simulink model "NL_Before_PLA"  (R2019b)
settings: Solver=VariableStepAuto  StartTime=0.0  StopTime=testtime  RelTol=1e-3
InitFcn:
  | NL_Before_PLA_Test_Parameters
StopFcn:
  | Verify_NL_Before_PLA
values from neighbouring files (symbols this model uses):
  cf_factor = min(cfsat, 10^(cfslope*cf/1e3 + cfconst)) * 2.0    [NL_Before_PLA_Test_Parameters.m]
  Fs = 48e3    (= 48000)    [NL_Before_PLA_Test_Parameters.m]
  multFac = max(2.95*max(1.0,1.5-spont/100), 4.3-0.2*cf/1e3)    [NL_Before_PLA_Test_Parameters.m]
  spont = 100    [NL_Before_PLA_Test_Parameters.m]
libraries: dspsrcs4 x2, simulink x1
settings Model: Creator=mblun  LastModifiedBy=t96f346
settings SFSimCC: CustomCodeUndefinedFunction=UseInterfaceOnly

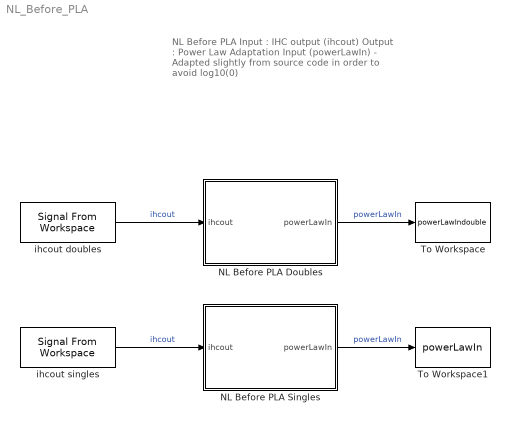
== system NL_Before_PLA ==
  note: NL Before PLA
      |
      | Input : IHC output (ihcout)
      |
      | Output : Power Law Adaptation Input (powerLawIn)
      |
      | - Adapted slightly from source code in order to avoid log10(0)
  NL Before PLA Doubles : Subsystem
  NL Before PLA Singles : Subsystem
  To Workspace : ToWorkspace  VariableName=powerLawIndouble  SampleTime=-1
      settings: Save2DSignal=2-D array (concatenate along first dimension)
  To Workspace1 : ToWorkspace  VariableName=powerLawIn  SampleTime=-1
      settings: Save2DSignal=2-D array (concatenate along first dimension)
  "ihcout doubles " : dspsrcs4/Signal From Workspace  X=RxSignalDouble  Ts=1/Fs  nsamps=1  OutputAfterFinalValue=Setting to zero  ignoreOrWarnInputAndFrameLengths=off  OutputFrames=off
  ihcout singles : dspsrcs4/Signal From Workspace  X=RxSignal  Ts=1/Fs  nsamps=1  OutputAfterFinalValue=Setting to zero  ignoreOrWarnInputAndFrameLengths=off  OutputFrames=off
  wires:
  NL Before PLA Doubles/1(powerLawIn) -> To Workspace/1  "powerLawIn"
  "ihcout doubles "/1 -> NL Before PLA Doubles/1(ihcout)  "ihcout"
  ihcout singles/1 -> NL Before PLA Singles/1(ihcout)  "ihcout"
  NL Before PLA Singles/1(powerLawIn) -> To Workspace1/1  "powerLawIn"

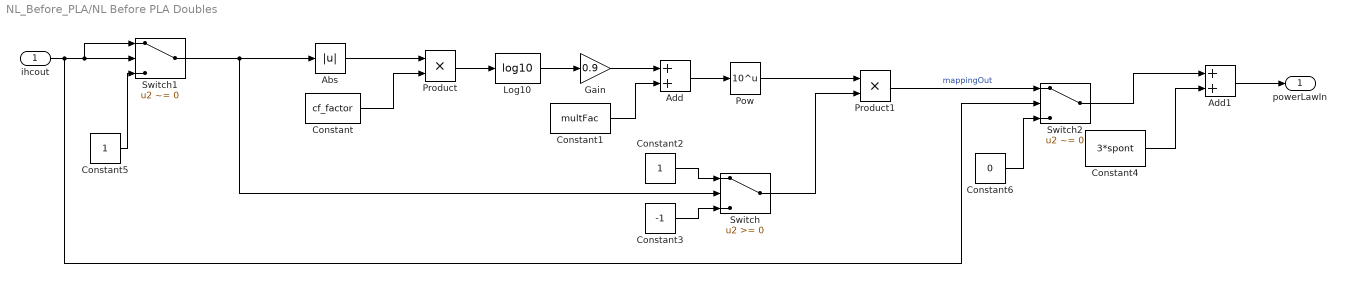
== system NL_Before_PLA/NL Before PLA Doubles ==
  ihcout : Inport
  Abs : Abs
  Add : Sum
  Add1 : Sum
  Constant : Constant  Value=cf_factor  SampleTime=-1
  Constant1 : Constant  Value=multFac  SampleTime=-1
  Constant2 : Constant  SampleTime=-1
  Constant3 : Constant  Value=-1  SampleTime=-1
  Constant4 : Constant  Value=3*spont  SampleTime=-1
  Constant5 : Constant  SampleTime=-1
  Constant6 : Constant  Value=0  SampleTime=-1
  Gain : Gain  Gain=0.9
  Log10 : Math  Operator=log10  RndMeth=Zero  SaturateOnIntegerOverflow=on
  Pow : Math  Operator=10^u  RndMeth=Zero  SaturateOnIntegerOverflow=on
  Product : Product
  Product1 : Product
  Switch : Switch
  Switch1 : Switch  Criteria=u2 ~= 0  ZeroCross=off
  Switch2 : Switch  Criteria=u2 ~= 0  ZeroCross=off
  powerLawIn : Outport  VectorParamsAs1DForOutWhenUnconnected=off
  wires:
  Switch1/1 -> Switch/2, Abs/1
  Constant/1 -> Product/2
  Abs/1 -> Product/1
  Product/1 -> Log10/1
  Log10/1 -> Gain/1
  Gain/1 -> Add/1
  Constant1/1 -> Add/2
  Add/1 -> Pow/1
  Constant3/1 -> Switch/3
  Constant2/1 -> Switch/1
  Pow/1 -> Product1/1
  Switch/1 -> Product1/2
  Constant4/1 -> Add1/2
  Add1/1 -> powerLawIn/1
  ihcout/1 -> Switch2/2, Switch1/1, Switch1/2
  Constant6/1 -> Switch2/3
  Switch2/1 -> Add1/1
  Constant5/1 -> Switch1/3
  Product1/1 -> Switch2/1  "mappingOut"

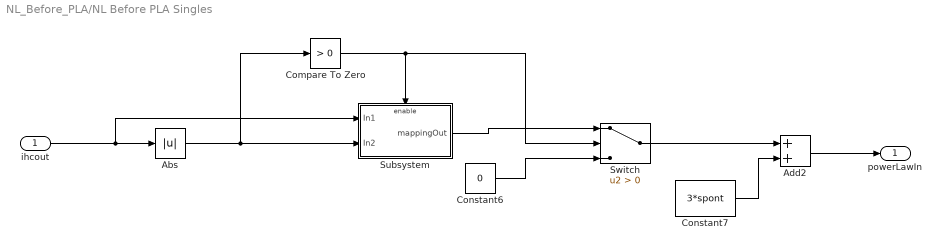
== system NL_Before_PLA/NL Before PLA Singles ==
  ihcout : Inport
  Abs : Abs
  Add2 : Sum
  Compare To Zero : simulink/Logic and Bit Operations/Compare To Zero  relop=>  OutDataTypeStr=boolean
  Constant6 : Constant  Value=0  OutDataTypeStr=single  SampleTime=-1
  Constant7 : Constant  Value=3*spont  OutDataTypeStr=single  SampleTime=-1
  Subsystem : Subsystem
  Switch : Switch  Criteria=u2 > Threshold  OutDataTypeStr=single
  powerLawIn : Outport  VectorParamsAs1DForOutWhenUnconnected=off
  wires:
  Constant6/1 -> Switch/3
  Switch/1 -> Add2/1
  Constant7/1 -> Add2/2
  Add2/1 -> powerLawIn/1
  ihcout/1 -> Subsystem/1(In1), Abs/1
  Abs/1 -> Compare To Zero/1, Subsystem/2(In2)
  Subsystem/1(mappingOut) -> Switch/1
  Compare To Zero/1 -> Subsystem/Enable, Switch/2

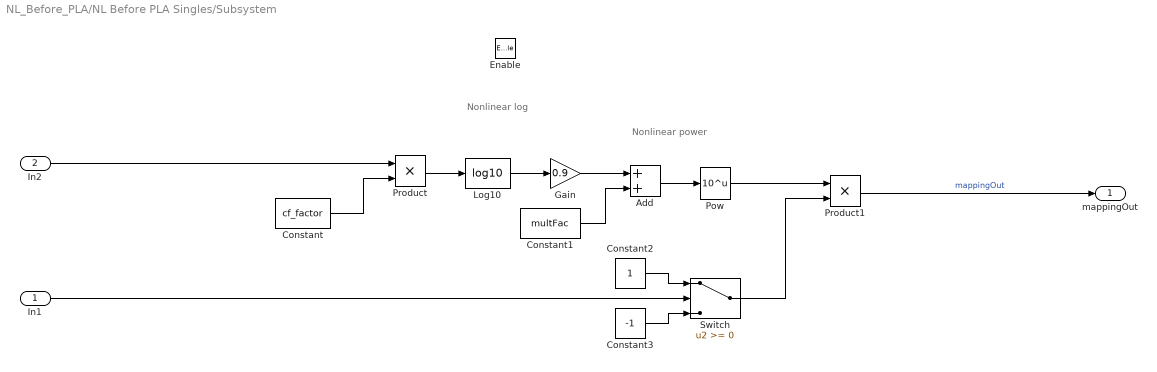
== system NL_Before_PLA/NL Before PLA Singles/Subsystem ==
  note: Nonlinear log
  note: Nonlinear power
  In1 : Inport
  In2 : Inport  Port=2
  Enable : EnablePort
  Add : Sum
  Constant : Constant  Value=cf_factor  OutDataTypeStr=single  SampleTime=-1
  Constant1 : Constant  Value=multFac  OutDataTypeStr=single  SampleTime=-1
  Constant2 : Constant  OutDataTypeStr=single  SampleTime=-1
  Constant3 : Constant  Value=-1  OutDataTypeStr=single  SampleTime=-1
  Gain : Gain  Gain=0.9
  Log10 : Math  Operator=log10  RndMeth=Zero  SaturateOnIntegerOverflow=on
  Pow : Math  Operator=10^u  RndMeth=Zero  SaturateOnIntegerOverflow=on
  Product : Product
  Product1 : Product
  Switch : Switch
  mappingOut : Outport
  wires:
  Constant3/1 -> Switch/3
  Switch/1 -> Product1/2
  Pow/1 -> Product1/1
  In1/1 -> Switch/2
  Constant/1 -> Product/2
  Product/1 -> Log10/1
  Constant2/1 -> Switch/1
  Log10/1 -> Gain/1
  Gain/1 -> Add/1
  Add/1 -> Pow/1
  Constant1/1 -> Add/2
  In2/1 -> Product/1
  Product1/1 -> mappingOut/1  "mappingOut"
